simulink model "NeuroSwarm"  (R2024b)
settings: Solver=VariableStepAuto  StartTime=0.0  StopTime=10  RelTol=1e-3
libraries: neural x32
(part 2 of 2)

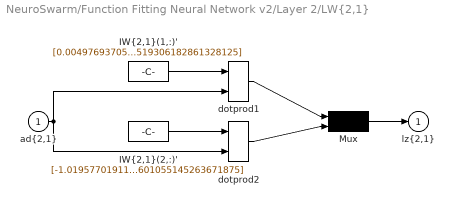
== system NeuroSwarm/Function Fitting Neural Network v2/Layer 2/LW{2,1} ==
  "ad{2,1}" : Inport  PortDimensions=10
      mask Display: e = 0.06;c1 = [120 230 180]/255;c2 = ([120 230 180]+0)/(256+128);c3 = ([120 230 180]+128)/(256+128);patch([0 1 1 0],[0 0 1 1],c1);patch([0 1 1 1-e 1-e 0+e],[0 0 1 1-e 0+e 0+e],c2);patch([0 0 1 1-e 0+e 0+e],[0 1 1 1-e 1-e 0+e],c3);plot([0 1 1 0 0],[0 0 1 1 0]);
  "IW{2,1}(1,:)'" : Constant  Value=[0.004976937054889675991764530493810525513254106044769287109375;2.231746101219425515438388174516148865222930908203125;-0.2717454779821364407865758039406500756740570068359375;20.585644582511985589690084452740848064422607421875;0.011016200715956388223037976104023982770740985870361328125;75.4182040659382124658804968930780887603759765625;-1.853508061759792990841333448770456016063690185546875;-1.806486775820502987954796481062658131122589111328125;-0.0139675176148385260521678219447494484484195709228515625;76.446001475737176633629132993519306182861328125]
      mask Display: e = 0.06;c1 = [120 150 230]/255;c2 = ([120 150 230]+0)/383;c3 = ([120 150 230]+128)/383;patch([0 1 1 0],[0 0 1 1],c1);patch([0 1 1 1-e 1-e 0+e],[0 0 1 1-e 0+e 0+e],c2);patch([0 0 1 1-e 0+e 0+e],[0 1 1 1-e 1-e 0+e],c3);plot([0 1 1 0 0],[0 0 1 1 0]);disp('weights');
  "IW{2,1}(2,:)'" : Constant  Value=[-1.019577019117841931716839098953641951084136962890625;0.0192327297271198717487639129331000731326639652252197265625;-51.61546278548248523065922199748456478118896484375;0.0347786257964664280439848198511754162609577178955078125;-16.11436728804136464532348327338695526123046875;-0.254269686168878461529629930737428367137908935546875;-48.3976878191570420995049062184989452362060546875;-95.9475484571545820244864444248378276824951171875;17.085678060315586890283157117664813995361328125;-0.25008468939349881576816869710455648601055145263671875]
      mask Display: e = 0.06;c1 = [120 150 230]/255;c2 = ([120 150 230]+0)/383;c3 = ([120 150 230]+128)/383;patch([0 1 1 0],[0 0 1 1],c1);patch([0 1 1 1-e 1-e 0+e],[0 0 1 1-e 0+e 0+e],c2);patch([0 0 1 1-e 0+e 0+e],[0 1 1 1-e 1-e 0+e],c3);plot([0 1 1 0 0],[0 0 1 1 0]);disp('weights');
  Mux : Mux  Inputs=2
      mask Display: e = 0.06;c1 = [120 150 230]/255;c2 = ([120 150 230]+0)/383;c3 = ([120 150 230]+128)/383;patch([0 1 1 0],[0 0 1 1],c1);patch([0 1 1 1-e 1-e 0+e],[0 0 1 1-e 0+e 0+e],c2);patch([0 0 1 1-e 0+e 0+e],[0 1 1 1-e 1-e 0+e],c3);plot([0 1 1 0 0],[0 0 1 1 0]);disp('Mux');
  dotprod1 : neural/Weight Functions/dotprod
  dotprod2 : neural/Weight Functions/dotprod
  "lz{2,1}" : Outport
      mask Display: e = 0.06;c1 = [120 230 180]/255;c2 = ([120 230 180]+0)/(256+128);c3 = ([120 230 180]+128)/(256+128);patch([0 1 1 0],[0 0 1 1],c1);patch([0 1 1 1-e 1-e 0+e],[0 0 1 1-e 0+e 0+e],c2);patch([0 0 1 1-e 0+e 0+e],[0 1 1 1-e 1-e 0+e],c3);plot([0 1 1 0 0],[0 0 1 1 0]);
  wires:
  "IW{2,1}(1,:)'"/1 -> dotprod1/1
  "ad{2,1}"/1 -> dotprod1/2, dotprod2/2
  dotprod1/1 -> Mux/1
  "IW{2,1}(2,:)'"/1 -> dotprod2/1
  dotprod2/1 -> Mux/2
  Mux/1 -> "lz{2,1}"/1

== matlab function NeuroSwarm/DEMUX ==
  data: u input; y1 output; y2 output
function [y1,y2] = fcn(u)

y1 = u(1);
y2 = u(2);

== matlab function NeuroSwarm/Mod ==
  data: q_1 input; truncq_1 output; q_2 input; truncq_2 output
function [truncq_1,truncq_2] = Truncation(q_1,q_2)

truncq_1 = mod( q_1 + pi, 2 * pi ) - pi;
truncq_2 = mod( q_2 + pi, 2 * pi ) - pi;
